simulink model "simulation_simconnect"  (R2020b)
settings: Solver=FixedStepAuto  StartTime=0.0  StopTime=inf  RelTol=1e-3
libraries: SimConnectToolbox x3, aerolibanimutils x1
settings Model: Creator=Andreas  LastModifiedBy=Andreas

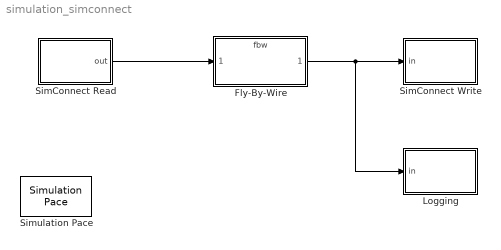
== system simulation_simconnect ==
  Fly-By-Wire : ModelReference  ModelNameDialog=fbw  ModelReferenceVersion=1.26
  Logging : Subsystem
  SimConnect Read : Subsystem
  SimConnect Write : Subsystem
  Simulation Pace : aerolibanimutils/Simulation Pace  SimulationPace=1  SleepMode=Auto  OutputPaceError=off  SampleTime=1/50
      settings: AttributesFormatString=%<SampleTime>
  wires:
  SimConnect Read/1(out) -> Fly-By-Wire/1
  Fly-By-Wire/1 -> Logging/1(in), SimConnect Write/1(in)

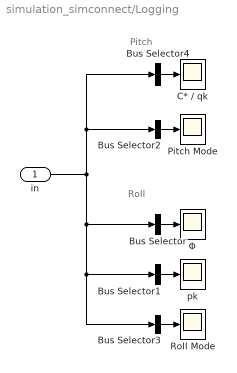
== system simulation_simconnect/Logging ==
  note: Pitch
  note: Roll
  in : Inport
  Bus Selector : BusSelector  OutputSignals=roll.roll:normal.Phi_c_deg,sim.sim:data.Phi_deg  OutputAsBus=on
  Bus Selector1 : BusSelector  OutputSignals=roll.roll:normal.pk_c_deg_s,sim.sim:data.pk_deg_s  OutputAsBus=on
  Bus Selector2 : BusSelector  OutputSignals=sim.sim:data:computed.on_ground,pitch.pitch:data:computed.in_flight,pitch.pitch:data:computed.in_flare,pitch.pitch:data:computed.in_flight_gain  OutputAsBus=on
  Bus Selector3 : BusSelector  OutputSignals=sim.sim:data:computed.on_ground,roll.roll:data:computed.in_flight,roll.roll:data:computed.in_flight_gain  OutputAsBus=on
  Bus Selector4 : BusSelector  OutputSignals=pitch.pitch:normal.Cstar_c_g,pitch.pitch:normal.Cstar_g,sim.sim:data.nz_g,sim.sim:data.qk_deg_s  OutputAsBus=on
  C* / qk : Scope
  Pitch Mode : Scope
  Roll Mode : Scope
  pk : Scope
  Φ : Scope
  wires:
  Bus Selector4/1 -> C* / qk/1
  Bus Selector1/1 -> pk/1
  Bus Selector/1 -> Φ/1
  in/1 -> Bus Selector4/1, Bus Selector2/1, Bus Selector1/1, Bus Selector3/1, Bus Selector/1
  Bus Selector2/1 -> Pitch Mode/1
  Bus Selector3/1 -> Roll Mode/1

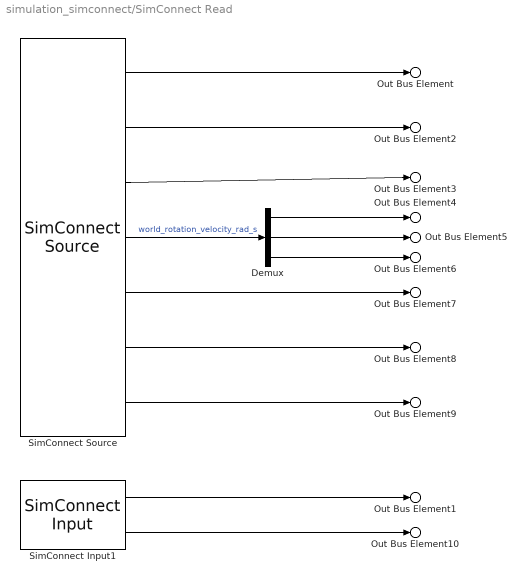
== system simulation_simconnect/SimConnect Read ==
  Demux : Demux  Outputs=3
  SimConnect Input1 : SimConnectToolbox/SimConnect Input  configurationIndex=0  connectionName=SimConnectInput_Pitch  variables=|
      | AXIS_ELEVATOR_SET, TRUE;
      | AXIS_AILERONS_SET, TRUE;
      settings: SourceProductName=SimConnect Toolbox
  SimConnect Source : SimConnectToolbox/SimConnect Source  configurationIndex=0  connectionName=SimConnectSource_Pitch  variables=|
      | G FORCE, GFORCE;
      | PLANE PITCH DEGREES, DEGREE;
      | PLANE BANK DEGREES, DEGREE;
      | STRUCT WORLD ROTATION VELOCITY, STRUCT;
      | AIRSPEED INDICATED, KNOTS;
      | RADIO HEIGHT, FEET;
      | CG PERCENT, PERCENT OVER 100;
      settings: SourceProductName=SimConnect Toolbox
  Out Bus Element : Outport  PortName=out  Element=sim.sim:raw:data.nz_g
  Out Bus Element2 : Outport  PortName=out  Element=sim.sim:raw:data.Theta_deg
  Out Bus Element3 : Outport  PortName=out  Element=sim.sim:raw:data.Phi_deg
  Out Bus Element4 : Outport  PortName=out  Element=sim.sim:raw:data.qk_rad_s
  Out Bus Element5 : Outport  PortName=out  Element=sim.sim:raw:data.rk_rad_s
  Out Bus Element6 : Outport  PortName=out  Element=sim.sim:raw:data.pk_rad_s
  Out Bus Element7 : Outport  PortName=out  Element=sim.sim:raw:data.Vk_kt
  Out Bus Element8 : Outport  PortName=out  Element=sim.sim:raw:data.radio_height_ft
  Out Bus Element9 : Outport  PortName=out  Element=sim.sim:raw:data.CG_percent_MAC
  Out Bus Element1 : Outport  PortName=out  Element=sim.sim:raw:input.delta_eta_pos
  Out Bus Element10 : Outport  PortName=out  Element=sim.sim:raw:input.delta_xi_pos
  wires:
  SimConnect Source/2 -> Out Bus Element2/1
  SimConnect Source/1 -> Out Bus Element/1
  SimConnect Source/3 -> Out Bus Element3/1
  SimConnect Source/4 -> Demux/1  "world_rotation_velocity_rad_s"
  SimConnect Source/5 -> Out Bus Element7/1
  SimConnect Source/6 -> Out Bus Element8/1
  SimConnect Source/7 -> Out Bus Element9/1
  SimConnect Input1/2 -> Out Bus Element10/1
  SimConnect Input1/1 -> Out Bus Element1/1
  Demux/1 -> Out Bus Element4/1
  Demux/2 -> Out Bus Element5/1
  Demux/3 -> Out Bus Element6/1

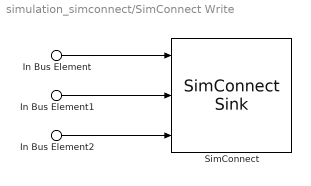
== system simulation_simconnect/SimConnect Write ==
  In Bus Element : Inport  PortName=in  Element=sim.sim:raw:output.eta_pos
  In Bus Element1 : Inport  PortName=in  Element=sim.sim:raw:output.iH_deg
  In Bus Element2 : Inport  PortName=in  Element=sim.sim:raw:output.xi_pos
  SimConnect : SimConnectToolbox/SimConnect Sink  configurationIndex=0  connectionName=SimConnectSink  variables=|
      | ELEVATOR POSITION, POSITION;
      | ELEVATOR TRIM POSITION, DEGREE;
      | AILERON POSITION, POSITION;
      settings: SourceProductName=SimConnect Toolbox
  wires:
  In Bus Element/1 -> SimConnect/1
  In Bus Element1/1 -> SimConnect/2
  In Bus Element2/1 -> SimConnect/3
